simulink model "sampleModel1777_2_sub_sub_sub"  (R2023a)
settings: Solver=VariableStepAuto  StartTime=0.0  StopTime=10.0  RelTol=1e-3
libraries: hdlsllib x4, simulink x2
settings Model: Creator=user1  LastModifiedBy=user1
settings OptimizationCC: BlockReduction=off  ConditionallyExecuteInputs=off

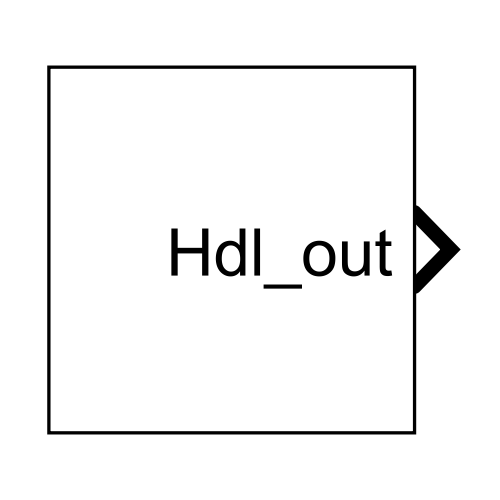
[thumbnail: Simulink's stored preview of the top-level diagram]
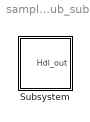
== system sampleModel1777_2_sub_sub_sub ==
  Subsystem : Subsystem

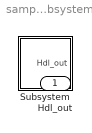
== system sampleModel1777_2_sub_sub_sub/Subsystem ==
  Subsystem : Subsystem
  Hdl_out : Outport  OutDataTypeStr=uint8

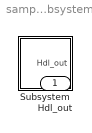
== system sampleModel1777_2_sub_sub_sub/Subsystem/Subsystem ==
  Subsystem : Subsystem
  Hdl_out : Outport  OutDataTypeStr=uint8

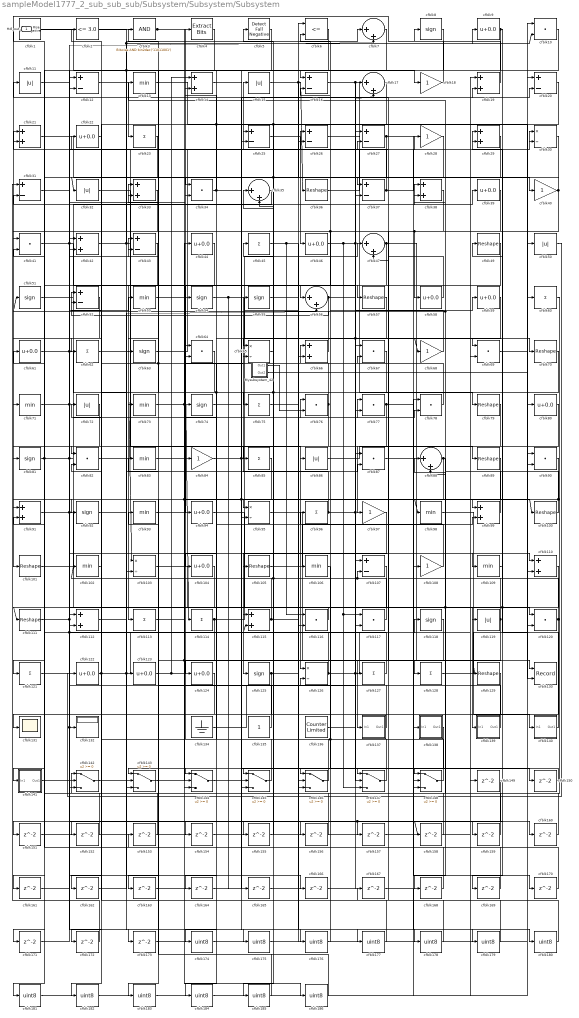
== system sampleModel1777_2_sub_sub_sub/Subsystem/Subsystem/Subsystem ==
  Mysubsystem_42 : Subsystem  TreatAsAtomicUnit=on  RTWFcnName=Mysubsystem_42
      settings: RTWFcnNameOpts=User specified  RTWFileNameOpts=Use function name
  cfblk1 : hdlsllib/Logic and Bit Operations/Detect Rise Nonnegative  vinit=0  OutDataTypeStr=uint8
  cfblk{10,34,41,64,67,69,76..78,82,87,90,116..117,120} (15 alike) : DotProduct  OutDataTypeStr=uint8
  cfblk{36,49,57,70,79,89,100..101,105,111,129} (11 alike) : Reshape
  cfblk{13,53,71,73,83,93,98,102,106,109} (10 alike) : MinMax  OutDataTypeStr=uint8
  cfblk{30,65,95,103,126} (5 alike) : Product  Inputs=*/  OutDataTypeStr=uint8  RndMeth=Zero  SaturateOnIntegerOverflow=on
  cfblk{9,22,39,44,46,58..59,61,80,94,104,122..124} (14 alike) : Bias  Bias=0.0  SaturateOnIntegerOverflow=off
  cfblk{12,16,20,25..27,31,37,43,52,107} (11 alike) : Sum  Inputs=+-  OutDataTypeStr=uint8
  cfblk{18,28,40,68,84,97,108} (7 alike) : Gain  OutDataTypeStr=uint8
  cfblk{11,15,32,50,72,86,119} (7 alike) : Abs  OutDataTypeStr=uint8  SaturateOnIntegerOverflow=off
  cfblk{14,19,21,29,33,38,42,66,91,99,110,112,115} (13 alike) : Sum  OutDataTypeStr=uint8
  cfblk{23,45,60,62,75,85,96,113..114,121,127..128} (12 alike) : Sum  Inputs=+  OutDataTypeStr=uint8
  cfblk{8,51,54..55,63,74,81,92,118,125} (10 alike) : Signum
  cfblk130 : Record  FileSettingsInternal="{\"entries\":[{\"content\":{\"excelSettings\":{\"content\":{},\"type\":\"Streamout.ExcelSettings\"}},\"type\":\"Streamout.FileSettingStorage\",\"uuid\":\"\"}],\"packageUris\":[\"http:\\/\\/schema.mathworks.com\\/mf0\\/streamout_blocks\\/R2020a\"],\"version\":\"1.0\"}"  Layout=[1 1]  SignalsInternal="{\"entries\":[{\"content\":{\"signals\":[{\"content\":{\"blockPath\":[],\"dimensions\":[1],\"domain\":\"\",\"lineColor\":\"#a2142f\",\"plots\":[1],\"port\":1,\"signalID\":41282,\"signalName\":\"cfblk47\"},\"type\":\"RecordBlkView.Signal\",\"uuid\":\"\"},{\"content\":{\"blockPath\":[],\"dimensions\":[1],\"domain\":\"\",\"lineColor\":\"#139fff\",\"plots\":[1],\"port\":2,\"signalID\":41285,\"signalName\":\"cfblk24\"},\"type\":\"RecordBlkView.Signal\",\"uuid\":\"\"}]},\"type\":\"RecordBlkView.InputSignals\",\"uuid\":\"\"}],\"packageUris\":[\"http:\\/\\/schema.mathworks.com\\/mf0\\/streamout_blocks\\/R2020a\"],\"version\":\"1.0\"}"  VisualizationBindings="{\"xyplotplugin\":{\"info\":[{\"series\":[{\"bindingParametersList\":[{\"parameter\":\"X-Axis\",\"signalID\":41282,\"signalName\":\"cfblk47\"},{\"parameter\":\"Y-Axis\",\"signalID\":41285,\"signalName\":\"cfblk24\"}],\"seriesID\":50401}],\"subplotID\":1}]}}"  CompatibilityTag=XY  st=-1
  cfblk131 : Scope
  cfblk132 : Display
  cfblk134 : Ground
  cfblk135 : Constant  OutDataTypeStr=uint8  SampleTime=-1
  cfblk136 : hdlsllib/Sources/Counter Limited  uplimit=7  tsamp=-1
  cfblk137 : Subsystem
      settings: LibrarySourceBlock=|
      | hdlsllib/Ports &
      | Subsystems/Subsystem
  cfblk138 : Subsystem
      settings: LibrarySourceBlock=|
      | hdlsllib/Ports &
      | Subsystems/Subsystem
  cfblk139 : Subsystem
      settings: LibrarySourceBlock=|
      | hdlsllib/Ports &
      | Subsystems/Subsystem
  cfblk140 : Subsystem
      settings: LibrarySourceBlock=|
      | hdlsllib/Ports &
      | Subsystems/Subsystem
  cfblk141 : Subsystem
      settings: LibrarySourceBlock=|
      | hdlsllib/Ports &
      | Subsystems/Subsystem
  cfblk{142..148} (7 alike) : Switch  OutDataTypeStr=uint8  SaturateOnIntegerOverflow=off  InputSameDT=off
  cfblk{149..173} (25 alike) : Delay  SampleTime=1
  cfblk{7,17,35,47,56,88} (6 alike) : Sum  Inputs=|++  OutDataTypeStr=uint8
  cfblk{174..186} (13 alike) : DataTypeConversion  OutDataTypeStr=uint8  SaturateOnIntegerOverflow=off  RndMeth=Floor
  cfblk2 : hdlsllib/Logic and Bit Operations/Compare To Constant  relop=<=  const=3.0  OutDataTypeStr=uint8
  cfblk3 : simulink/Logic and Bit Operations/Bitwise Operator  logicop=AND  UseBitMask=on  BitMask=bin2dec('11011001')  BitMaskRealWorld=Stored Integer
      settings: LibrarySourceBlock=|
      | hdlsllib/Logic and Bit
      | Operations/Bitwise
      | Operator
  cfblk4 : simulink/Logic and Bit Operations/Extract Bits  bitsToExtract=Upper half  numBits=8  bitIdxRange=[0 7]  outScalingMode=Preserve fixed-point scaling
      settings: LibrarySourceBlock=|
      | hdlsllib/Logic and Bit
      | Operations/Extract Bits
  cfblk5 : hdlsllib/Logic and Bit Operations/Detect Fall Negative  vinit=0  OutDataTypeStr=uint8
  cfblk6 : RelationalOperator  Operator=<=  OutDataTypeStr=boolean  InputSameDT=off
  Hdl_out : Outport  OutDataTypeStr=uint8
  wires:
  cfblk147/1 -> cfblk4/1
  cfblk54/1 -> cfblk165/1, cfblk70/1
  cfblk62/1 -> cfblk30/1
  cfblk25/1 -> cfblk46/1
  cfblk19/1 -> cfblk101/1
  cfblk60/1 -> cfblk142/1
  cfblk50/1 -> cfblk122/1
  cfblk98/1 -> cfblk140/1(In1)
  cfblk44/1 -> cfblk113/1
  cfblk58/1 -> cfblk11/1
  cfblk80/1 -> cfblk97/1
  cfblk16/1 -> cfblk69/1, cfblk79/1
  cfblk52/1 -> cfblk71/1
  cfblk70/1 -> cfblk164/1, cfblk114/1
  cfblk49/1 -> cfblk94/1
  cfblk63/1 -> cfblk20/1
  cfblk39/1 -> cfblk142/3, cfblk56/1
  cfblk47/1 -> cfblk57/1, cfblk130/1
  cfblk79/1 -> cfblk126/1
  cfblk103/1 -> cfblk139/1(In1)
  cfblk53/1 -> cfblk15/1
  cfblk121/1 -> cfblk126/2
  cfblk129/1 -> cfblk131/1
  cfblk42/1 -> cfblk86/1, cfblk7/1, cfblk10/2
  cfblk51/1 -> cfblk38/1
  cfblk9/1 -> cfblk159/1, cfblk16/1
  cfblk101/1 -> cfblk39/1
  cfblk89/1 -> cfblk95/2, cfblk143/1
  cfblk119/1 -> cfblk88/1, cfblk124/1
  cfblk141/1(Out1) -> cfblk132/1, cfblk7/2, cfblk115/2
  cfblk57/1 -> cfblk144/1
  cfblk17/1 -> cfblk65/1, cfblk34/1
  cfblk13/1 -> cfblk80/1
  cfblk145/1 -> cfblk64/1
  cfblk91/1 -> cfblk34/2, cfblk119/1
  cfblk95/1 -> cfblk137/1(In1)
  cfblk27/1 -> cfblk99/1, cfblk75/1, cfblk32/1
  cfblk12/1 -> cfblk23/1
  cfblk97/1 -> cfblk125/1
  cfblk148/1 -> cfblk82/2, cfblk96/1
  cfblk87/1 -> cfblk120/1
  cfblk100/1 -> cfblk98/1, cfblk13/1, cfblk51/1
  cfblk81/1 -> cfblk41/2, cfblk116/2, cfblk76/1
  cfblk72/1 -> cfblk142/2
  cfblk143/1 -> cfblk118/1
  cfblk114/1 -> cfblk163/1, cfblk47/1
  cfblk127/1 -> cfblk61/1
  cfblk15/1 -> cfblk37/2, cfblk36/1
  cfblk82/1 -> cfblk28/1
  cfblk111/1 -> cfblk160/1, cfblk43/2
  cfblk122/1 -> cfblk52/1, cfblk56/2, cfblk67/1
  cfblk76/1 -> cfblk121/1, cfblk22/1, cfblk33/1
  cfblk93/1 -> cfblk44/1
  cfblk71/1 -> cfblk173/1, cfblk53/1
  cfblk142/1 -> cfblk158/1, cfblk157/1
  cfblk67/1 -> cfblk95/1, cfblk103/1
  cfblk139/1(Out1) -> cfblk93/1
  cfblk128/1 -> cfblk10/1
  cfblk59/1 -> cfblk145/1
  cfblk96/1 -> cfblk55/1, cfblk128/1, cfblk17/2
  cfblk40/1 -> cfblk37/1, cfblk127/1, cfblk58/1
  cfblk36/1 -> cfblk30/2
  cfblk105/1 -> cfblk17/1
  cfblk23/1 -> cfblk112/2
  cfblk108/1 -> cfblk74/1
  cfblk109/1 -> cfblk49/1
  cfblk1/1 -> cfblk18/1
  cfblk90/1 -> cfblk91/1
  cfblk21/1 -> cfblk108/1
  cfblk77/1 -> cfblk170/1, cfblk141/1(In1), cfblk84/1
  cfblk37/1 -> cfblk29/2, cfblk21/1
  cfblk86/1 -> cfblk89/1
  cfblk7/1 -> cfblk145/2
  cfblk61/1 -> cfblk105/1, cfblk123/1
  cfblk35/1 -> cfblk31/2
  cfblk140/1(Out1) -> cfblk29/1
  cfblk126/1 -> cfblk21/2, cfblk99/2, cfblk69/2
  cfblk84/1 -> cfblk110/2, cfblk9/1
  cfblk116/1 -> cfblk115/1
  cfblk41/1 -> cfblk166/1, cfblk54/1
  cfblk146/1 -> cfblk35/2
  cfblk106/1 -> cfblk146/1
  cfblk99/1 -> cfblk38/2
  cfblk8/1 -> cfblk12/2
  cfblk4/1 -> cfblk63/1
  cfblk115/1 -> cfblk180/1, cfblk33/2
  cfblk55/1 -> cfblk106/1
  cfblk45/1 -> cfblk116/1, cfblk109/1
  cfblk11/1 -> cfblk42/1
  cfblk134/1 -> cfblk87/1
  cfblk28/1 -> cfblk62/1
  cfblk125/1 -> cfblk144/3, cfblk77/1
  cfblk94/1 -> cfblk120/2
  cfblk88/1 -> cfblk146/3, cfblk148/1
  cfblk38/1 -> cfblk73/1
  cfblk30/1 -> cfblk144/2
  cfblk113/1 -> cfblk78/2
  cfblk83/1 -> cfblk117/2, cfblk100/1
  cfblk43/1 -> cfblk81/1
  cfblk123/1 -> cfblk14/1, cfblk129/1, cfblk64/2
  cfblk66/1 -> cfblk5/1
  cfblk137/1(Out1) -> cfblk83/1
  cfblk56/1 -> cfblk52/2, cfblk68/1, cfblk107/1
  cfblk110/1 -> cfblk169/1, cfblk168/1, cfblk111/1
  cfblk120/1 -> cfblk47/2, cfblk145/3
  cfblk92/1 -> cfblk87/2
  cfblk20/1 -> cfblk104/1, cfblk82/1
  cfblk34/1 -> cfblk14/2, cfblk20/2
  cfblk117/1 -> cfblk107/2, cfblk45/1, cfblk102/1
  cfblk68/1 -> cfblk26/1
  cfblk78/1 -> cfblk66/1
  cfblk32/1 -> cfblk147/2
  cfblk136/1 -> cfblk59/1
  cfblk73/1 -> cfblk65/2, cfblk85/1
  cfblk46/1 -> cfblk110/1, cfblk27/1, cfblk147/3, cfblk117/1
  cfblk135/1 -> cfblk43/1
  cfblk10/1 -> cfblk143/3, cfblk41/1
  cfblk26/1 -> cfblk40/1
  cfblk75/1 -> cfblk19/2
  cfblk31/1 -> cfblk25/1
  cfblk22/1 -> cfblk92/1
  cfblk18/1 -> cfblk8/1
  cfblk69/1 -> cfblk60/1
  cfblk144/1 -> cfblk150/1
  cfblk150/1 -> cfblk147/1
  cfblk104/1 -> cfblk151/1
  cfblk151/1 -> cfblk78/1
  cfblk107/1 -> cfblk152/1
  cfblk152/1 -> cfblk112/1
  cfblk153/1 -> cfblk143/2
  cfblk85/1 -> cfblk154/1
  cfblk65/1 -> cfblk155/1
  cfblk155/1 -> cfblk35/1
  cfblk74/1 -> cfblk156/1
  cfblk156/1 -> cfblk146/2
  cfblk157/1 -> cfblk19/1
  cfblk158/1 -> cfblk16/2
  cfblk159/1 -> cfblk88/2
  cfblk160/1 -> cfblk1/1
  cfblk33/1 -> cfblk161/1
  cfblk161/1 -> cfblk42/2
  cfblk64/1 -> cfblk162/1
  cfblk162/1 -> cfblk103/2
  cfblk163/1 -> cfblk26/2
  cfblk164/1 -> cfblk25/2
  cfblk165/1 -> cfblk77/2
  cfblk166/1 -> cfblk148/3
  cfblk168/1 -> cfblk148/2
  cfblk169/1 -> cfblk27/2
  cfblk170/1 -> cfblk91/2
  cfblk29/1 -> cfblk171/1
  cfblk171/1 -> cfblk12/1
  cfblk102/1 -> cfblk172/1
  cfblk172/1 -> cfblk31/1
  cfblk173/1 -> cfblk66/2
  cfblk6/1 -> cfblk174/1
  cfblk174/1 -> cfblk50/1
  cfblk112/1 -> cfblk175/1
  cfblk175/1 -> cfblk6/1
  cfblk154/1 -> cfblk176/1
  cfblk176/1 -> cfblk6/2
  cfblk2/1 -> cfblk177/1
  cfblk177/1 -> cfblk72/1
  cfblk14/1 -> cfblk178/1
  cfblk178/1 -> cfblk2/1
  cfblk167/1 -> cfblk179/1
  cfblk179/1 -> cfblk67/2
  cfblk180/1 -> cfblk167/1
  cfblk149/1 -> cfblk181/1
  cfblk181/1 -> cfblk90/1
  cfblk124/1 -> cfblk182/1
  cfblk182/1 -> cfblk149/1
  cfblk138/1(Out1) -> cfblk183/1
  cfblk183/1 -> cfblk90/2
  cfblk5/1 -> cfblk184/1
  cfblk184/1 -> cfblk138/1(In1)
  cfblk118/1 -> cfblk185/1
  cfblk185/1 -> cfblk3/1
  cfblk3/1 -> Hdl_out/1, cfblk186/1
  cfblk186/1 -> cfblk153/1
  Mysubsystem_42/1(Out1) -> cfblk76/2
  Mysubsystem_42/2(Out2) -> cfblk130/2

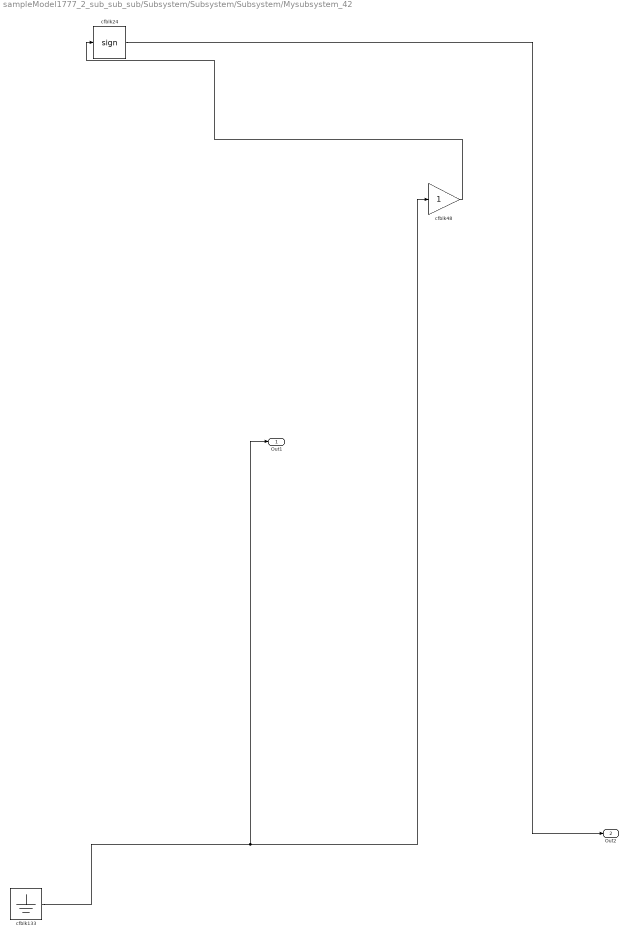
== system sampleModel1777_2_sub_sub_sub/Subsystem/Subsystem/Subsystem/Mysubsystem_42 ==
  cfblk133 : Ground
  cfblk24 : Signum
  cfblk48 : Gain
  Out1 : Outport
  Out2 : Outport  Port=2
  wires:
  cfblk24/1 -> Out2/1
  cfblk133/1 -> cfblk48/1, Out1/1
  cfblk48/1 -> cfblk24/1

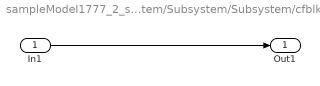
== system sampleModel1777_2_sub_sub_sub/Subsystem/Subsystem/Subsystem/cfblk137 ==
  In1 : Inport
  Out1 : Outport
  wires:
  In1/1 -> Out1/1

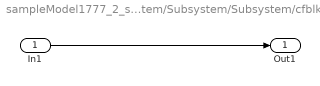
== system sampleModel1777_2_sub_sub_sub/Subsystem/Subsystem/Subsystem/cfblk138 ==
  In1 : Inport
  Out1 : Outport
  wires:
  In1/1 -> Out1/1

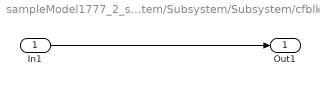
== system sampleModel1777_2_sub_sub_sub/Subsystem/Subsystem/Subsystem/cfblk139 ==
  In1 : Inport
  Out1 : Outport
  wires:
  In1/1 -> Out1/1

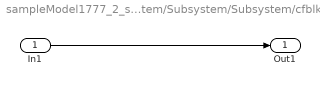
== system sampleModel1777_2_sub_sub_sub/Subsystem/Subsystem/Subsystem/cfblk140 ==
  In1 : Inport
  Out1 : Outport
  wires:
  In1/1 -> Out1/1

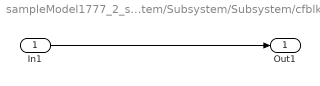
== system sampleModel1777_2_sub_sub_sub/Subsystem/Subsystem/Subsystem/cfblk141 ==
  In1 : Inport
  Out1 : Outport
  wires:
  In1/1 -> Out1/1
